simulink model "sync_mach_cont_sim"  (R2017a)
settings: Solver=ode23tb  StartTime=0.0  StopTime=10.0  FixedStep=1e-5  RelTol=1e-3
values from neighbouring files (symbols this model uses):
  L_1 = inv(L)    [smparamlib.m]
  Ra = .018    (= 0.018)    [smparamlib.m]
  Rf = 0.001    [smparamlib.m]
  Rkd = 0.02    [smparamlib.m]
  Rkq = 0.04    [smparamlib.m]
  wo = 2*pi*freq0    (= 376.991118431)    [smparamlib.m]
settings Model: Creator=krovchen  LastModifiedBy=krovchen
settings OptimizationCC: DefaultParameterBehavior=Inlined  UseDivisionForNetSlopeComputation=on  UseFloatMulNetSlope=on  InlineInvariantSignals=on  PassReuseOutputArgsThreshold=0  EfficientFloat2IntCast=on
settings DebuggingCC: ParameterTunabilityLossMsg=error
settings HardwareCC: TargetBitPerPointer=64  TargetBitPerSizeT=64  TargetBitPerPtrDiffT=64  TargetLongLongMode=on  TargetIntDivRoundTo=Zero  TargetEndianess=LittleEndian  TargetWordSize=64  TargetHWDeviceType=MATLAB Host  ProdEqTarget=off
settings SFSimCC: MATLABDynamicMemAlloc=off
settings RTWCC: SystemTargetFile=rsim.tlc  GenCodeOnly=on  PackageGeneratedCodeAndArtifacts=on  PackageName=v1_model_export  TemplateMakefile=rsim_default_tmf  Description=Rapid Simulation Target  GenerateReport=on  LaunchReport=on  TargetLang=C++
settings CodeAppCC: ForceParamTrailComments=on  OperatorAnnotations=on  MATLABSourceComments=on
settings RSimTargetCC: TargetLangStandard=C++03 (ISO)  GeneratePreprocessorConditionals=Use local settings

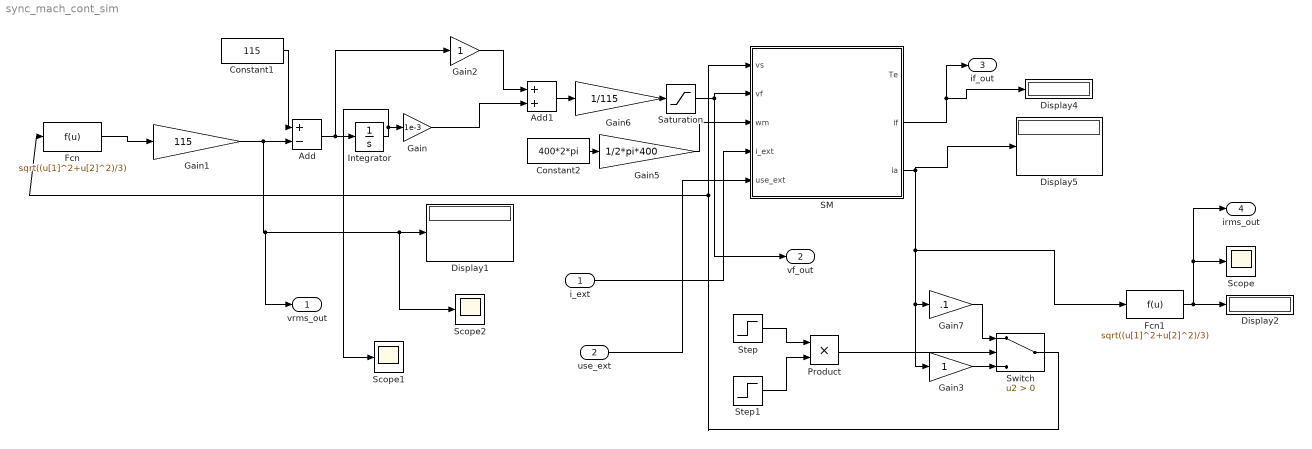
== system sync_mach_cont_sim ==
  i_ext : Inport
  use_ext : Inport  Port=2
  Add : Sum  Inputs=+-
  Add1 : Sum
  Constant1 : Constant  Value=115
  Constant2 : Constant  Value=400*2*pi
  Display{1..2,4..5} (4 alike) : Display
  Fcn : Fcn  Expr=sqrt((u[1]^2+u[2]^2)/3)
  Fcn1 : Fcn  Expr=sqrt((u[1]^2+u[2]^2)/3)
  Gain : Gain  Gain=1e-3
  Gain1 : Gain  Gain=115
  Gain2 : Gain
  Gain3 : Gain
  Gain5 : Gain  Gain=1/2*pi*400
  Gain6 : Gain  Gain=1/115
  Gain7 : Gain  Gain=.1
  Integrator : Integrator  LimitOutput=on  UpperSaturationLimit=1  LowerSaturationLimit=-1
  Product : Product
  SM : Subsystem
      mask Display:
      | plot(-1.5,-1.5,1.5,1.5,cos(0:.01:7),sin(0:.01:7),[-.5 -1 1 .5],[-.866 -1.2 -1.2 -.866] )
      | disp('SYNCHRONOUS\nMACHINE')
  Saturation : Saturate  UpperLimit=1  LowerLimit=-1
  Scope : Scope
  Scope1 : Scope
  Scope2 : Scope
  Step : Step  Time=5  SampleTime=0
  Step1 : Step  Time=7  Before=1  After=0  SampleTime=0
  Switch : Switch  Criteria=u2 > Threshold
  vrms_out : Outport
  vf_out : Outport  Port=2
  if_out : Outport  Port=3
  irms_out : Outport  Port=4
  wires:
  Constant2/1 -> Gain5/1
  Gain5/1 -> SM/3(wm)
  Add1/1 -> Gain6/1
  Gain6/1 -> Saturation/1
  Fcn/1 -> Gain1/1
  Gain1/1 -> vrms_out/1, Scope2/1, Display1/1, Add/2
  Constant1/1 -> Add/1
  Add/1 -> Gain2/1, Integrator/1
  Integrator/1 -> Scope1/1, Gain/1
  Gain/1 -> Add1/2
  Gain2/1 -> Add1/1
  SM/3(ia) -> Display5/1, Fcn1/1, Gain3/1, Gain7/1
  Fcn1/1 -> irms_out/1, Scope/1, Display2/1
  Step/1 -> Product/1
  Step1/1 -> Product/2
  Product/1 -> Switch/2
  Gain7/1 -> Switch/1
  Gain3/1 -> Switch/3
  Switch/1 -> Fcn/1, SM/1(vs)
  Saturation/1 -> vf_out/1, SM/2(vf)
  SM/2(if) -> if_out/1, Display4/1
  i_ext/1 -> SM/4(i_ext)
  use_ext/1 -> SM/5(use_ext)

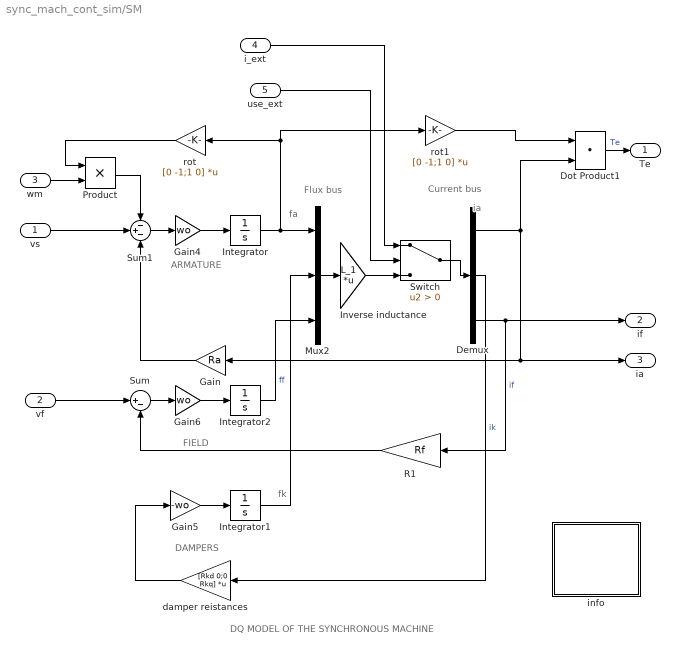
== system sync_mach_cont_sim/SM ==
  note: DAMPERS
  note: ARMATURE
  note: fa
  note: fk
  note: ia
  note: FIELD
  note: DQ MODEL OF THE SYNCHRONOUS MACHINE
  note: Flux bus
  note: Current bus
  vs : Inport
  vf : Inport  Port=2
  wm : Inport  Port=3
  i_ext : Inport  Port=4
  use_ext : Inport  Port=5
  Demux : Demux  Outputs=3
  Dot Product1 : DotProduct  InputSameDT=on  OutDataTypeStr=Inherit: Inherit via internal rule
  Gain : Gain  Gain=Ra  SaturateOnIntegerOverflow=on  OutDataTypeStr=Inherit: Same as input  ParamDataTypeStr=Inherit: Same as input
  Gain4 : Gain  Gain=wo  SaturateOnIntegerOverflow=on  OutDataTypeStr=Inherit: Same as input  ParamDataTypeStr=Inherit: Same as input
  Gain5 : Gain  Gain=-wo  SaturateOnIntegerOverflow=on  OutDataTypeStr=Inherit: Same as input  ParamDataTypeStr=Inherit: Same as input
  Gain6 : Gain  Gain=wo  SaturateOnIntegerOverflow=on  OutDataTypeStr=Inherit: Same as input  ParamDataTypeStr=Inherit: Same as input
  Integrator : Integrator  InitialCondition=[0 0]
  Integrator1 : Integrator  InitialCondition=[0 0]
  Integrator2 : Integrator
  Inverse inductance : Gain  Gain=L_1  Multiplication=Matrix(K*u)  SaturateOnIntegerOverflow=on  OutDataTypeStr=Inherit: Same as input  ParamDataTypeStr=Inherit: Same as input
  Mux2 : Mux  Inputs=3
  Product : Product  SaturateOnIntegerOverflow=on  InputSameDT=on  OutDataTypeStr=Inherit: Same as first input
  R1 : Gain  Gain=Rf  SaturateOnIntegerOverflow=on  OutDataTypeStr=Inherit: Same as input  ParamDataTypeStr=Inherit: Same as input
  Sum : Sum  Inputs=|+-  SaturateOnIntegerOverflow=on  InputSameDT=on  OutDataTypeStr=Inherit: Same as first input
  Sum1 : Sum  Inputs=-+-  SaturateOnIntegerOverflow=on  InputSameDT=on  OutDataTypeStr=Inherit: Same as first input
  Switch : Switch  Criteria=u2 > Threshold
  damper reistances : Gain  Gain=[Rkd 0;0 Rkq]  Multiplication=Matrix(K*u)  SaturateOnIntegerOverflow=on  OutDataTypeStr=Inherit: Same as input  ParamDataTypeStr=Inherit: Same as input
  info : Subsystem
      settings: OpenFcn=helpview(which('smeq0.htm'));
      mask Display:
      | plot(-1.5,-1.5,1.5,1.5,cos(0:.01:7),sin(0:.01:7) )
      | disp('Equations')
  rot : Gain  Gain=[0 -1;1 0]  Multiplication=Matrix(K*u)  SaturateOnIntegerOverflow=on  OutDataTypeStr=Inherit: Same as input  ParamDataTypeStr=Inherit: Same as input
  rot1 : Gain  Gain=[0 -1;1 0]  Multiplication=Matrix(K*u)  SaturateOnIntegerOverflow=on  OutDataTypeStr=Inherit: Same as input  ParamDataTypeStr=Inherit: Same as input
  Te : Outport
  if : Outport  Port=2
  ia : Outport  Port=3
  wires:
  Product/1 -> Sum1/1
  rot/1 -> Product/1
  wm/1 -> Product/2
  Gain5/1 -> Integrator1/1
  damper reistances/1 -> Gain5/1
  Integrator/1 -> Mux2/1, rot/1, rot1/1
  Sum1/1 -> Gain4/1
  Gain4/1 -> Integrator/1
  vs/1 -> Sum1/2
  Gain/1 -> Sum1/3
  Gain6/1 -> Integrator2/1
  Sum/1 -> Gain6/1
  vf/1 -> Sum/1
  rot1/1 -> Dot Product1/1
  Dot Product1/1 -> Te/1  "Te"
  Mux2/1 -> Inverse inductance/1
  Integrator1/1 -> Mux2/2
  Integrator2/1 -> Mux2/3  "ff"
  Demux/3 -> if/1, R1/1  "if"
  Demux/2 -> damper reistances/1  "ik"
  Inverse inductance/1 -> Switch/3
  Demux/1 -> Gain/1, ia/1, Dot Product1/2
  R1/1 -> Sum/2
  Switch/1 -> Demux/1
  use_ext/1 -> Switch/2
  i_ext/1 -> Switch/1

== system sync_mach_cont_sim/SM/info ==
  note: This  demonstration  illustrates  the dynamics of a synchronous generator, initially
      | at no load,  following a three-phase short circuit at the terminals.
  note: Synchronous machine transients
      | under shortcircuit
